simulink model "PowerWindowControl_V5"  (R2021a)
settings: Solver=VariableStepAuto  StartTime=0.0  StopTime=20  RelTol=1e-3
model workspace (MAT data in the model file):
  B = 0.01
  Ke_phi = 1.6
  Ra = 0.5
  TL = 20
  tau_a1 = 0.2
  tau_m = 500
settings Model: EnablePacing=on  PacingRate=0.630000  Creator=achu  LastModifiedBy=achu

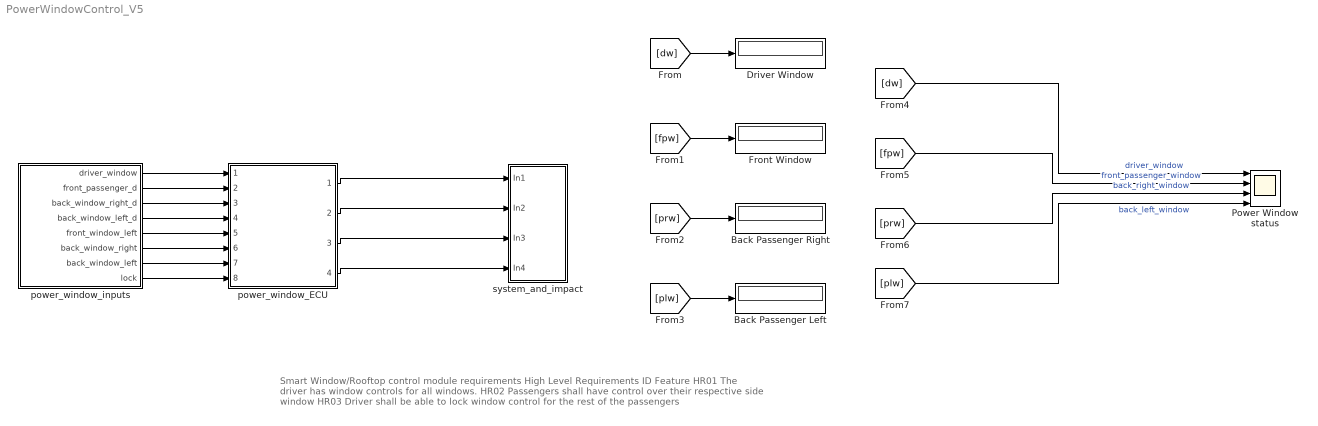
== system PowerWindowControl_V5 ==
  note: Smart Window/Rooftop control module requirements
      |
      | High Level Requirements
      |
      | ID
      | Feature
      |
      | HR01
      | The driver has window controls for all windows.
      |
      | HR02
      | Passengers shall have control over their respective side window
      |
      | HR03
      | Driver shall be able to lock window control for the rest of the passengers
  Back Passenger Left : Display
  Back Passenger Right : Display
  Driver Window : Display
  Front Window : Display
  Power Window status : Scope  NumInputPorts=4
  power_window_ECU : Subsystem  ReferencedSubsystem=power_window_ECU
  power_window_inputs : Subsystem
  system_and_impact : Subsystem
  wires:
  power_window_inputs/1(driver_window) -> power_window_ECU/1
  power_window_inputs/2(front_passenger_d) -> power_window_ECU/2
  power_window_inputs/3(back_window_right_d) -> power_window_ECU/3
  power_window_inputs/4(back_window_left_d) -> power_window_ECU/4
  power_window_inputs/5(front_window_left) -> power_window_ECU/5
  power_window_inputs/6(back_window_right) -> power_window_ECU/6
  power_window_inputs/7(back_window_left) -> power_window_ECU/7
  power_window_ECU/1 -> system_and_impact/1(In1)
  power_window_ECU/2 -> system_and_impact/2(In2)
  power_window_ECU/3 -> system_and_impact/3(In3)
  power_window_ECU/4 -> system_and_impact/4(In4)
  [prw] -> Back Passenger Right/1
  [dw] -> Power Window status/1  "driver_window"
  [prw] -> Power Window status/3  "back_right_window"
  [plw] -> Power Window status/4  "back_left_window"
  [fpw] -> Power Window status/2  "front_passenger_window"
  [plw] -> Back Passenger Left/1
  [fpw] -> Front Window/1
  [dw] -> Driver Window/1
  power_window_inputs/8(lock) -> power_window_ECU/8

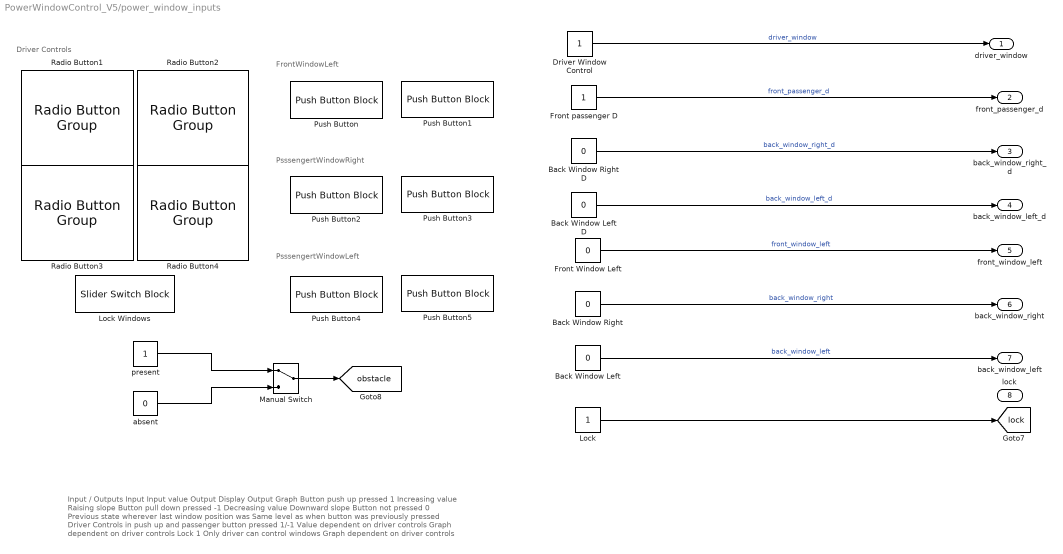
== system PowerWindowControl_V5/power_window_inputs ==
  note: PsssengertWindowLeft
  note: PsssengertWindowRight
  note: Driver Controls
  note: FrontWindowLeft
  note: Input / Outputs
      |
      | Input
      | Input value
      | Output Display
      | Output Graph
      |
      | Button push up pressed
      | 1
      | Increasing value
      | Raising slope
      |
      | Button pull down pressed
      | -1
      | Decreasing value
      | Downward slope
      |
      | Button not pressed
      | 0
      | Previous state wherever last window position was
      | Same level as when button was previously pressed
      |
      | Driver Controls in push up and passenger button pressed
      | 1/-1
      | Value dependent on driver controls
      | Graph dependent on driver controls
      |
      | Lock
      | 1
      | Only driver can control windows
      | Graph dependent on driver controls
  Back Window Left : Constant  Value=0
  Back Window Left D : Constant  Value=0
  Back Window Right : Constant  Value=0
  Back Window Right D : Constant  Value=0
  Driver Window Control : Constant
  Front Window Left : Constant  Value=0
  Front passenger D : Constant
  Lock : Constant
  Lock Windows : SliderSwitchBlock
      settings: Values={{'Unlock', 'Lock'}, [0 1]}
  Manual Switch : ManualSwitch
  Push Button : PushButtonBlock  ButtonText=Push up window
  Push Button1 : PushButtonBlock  ButtonText=Pull down window  OnValue=-1
  Push Button2 : PushButtonBlock  ButtonText=Push up window
  Push Button3 : PushButtonBlock  ButtonText=Pull down window  OnValue=-1
  Push Button4 : PushButtonBlock  ButtonText=Push up window
  Push Button5 : PushButtonBlock  ButtonText=Pull down window  OnValue=-1
  Radio Button1 : RadioButtonGroup  LabelPosition=Hide  SelectedLabel=Open  ButtonGroupName=Driver Window Controls
      settings: Values={{'Open', 'Stop', 'Close'}, [1 0 -1]}
  Radio Button2 : RadioButtonGroup  LabelPosition=Hide  SelectedLabel=Open  ButtonGroupName=Front Passenger
      settings: Values={{'Open', 'Stop', 'Close'}, [1 0 -1]}
  Radio Button3 : RadioButtonGroup  LabelPosition=Hide  SelectedLabel=Stop  ButtonGroupName=Back Window Right
      settings: Values={{'Open', 'Stop', 'Close'}, [1 0 -1]}
  Radio Button4 : RadioButtonGroup  LabelPosition=Hide  SelectedLabel=Stop  ButtonGroupName=Back Window Left
      settings: Values={{'Open', 'Stop', 'Close'}, [1 0 -1]}
  absent : Constant  Value=0
  present : Constant
  driver_window : Outport
  front_passenger_d : Outport  Port=2
  back_window_right_d : Outport  Port=3
  back_window_left_d : Outport  Port=4
  front_window_left : Outport  Port=5
  back_window_right : Outport  Port=6
  back_window_left : Outport  Port=7
  lock : Outport  Port=8
  tag scope: lock=global, obstacle=global
  wires:
  Front Window Left/1 -> front_window_left/1  "front_window_left"
  Front passenger D/1 -> front_passenger_d/1  "front_passenger_d"
  Back Window Right/1 -> back_window_right/1  "back_window_right"
  Back Window Left D/1 -> back_window_left_d/1  "back_window_left_d"
  Driver Window Control/1 -> driver_window/1  "driver_window"
  Back Window Left/1 -> back_window_left/1  "back_window_left"
  Back Window Right D/1 -> back_window_right_d/1  "back_window_right_d"
  Manual Switch/1 -> [obstacle]
  Lock/1 -> [lock]
  present/1 -> Manual Switch/1
  absent/1 -> Manual Switch/2

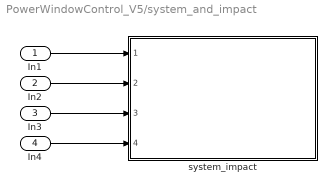
== system PowerWindowControl_V5/system_and_impact ==
  In1 : Inport
  In2 : Inport  Port=2
  In3 : Inport  Port=3
  In4 : Inport  Port=4
  system_impact : Subsystem  ReferencedSubsystem=power_window_system_impact
  wires:
  In4/1 -> system_impact/4
  In2/1 -> system_impact/2
  In3/1 -> system_impact/3
  In1/1 -> system_impact/1
